simulink model "simulink_computer_auto_highlighted"  (R2022b)
settings: Solver=VariableStepAuto  StartTime=0.0  StopTime=inf  RelTol=1e-3
libraries: simulink_extras x21, dspswit3 x1, simulink x1, hdlsllib x1
(part 2 of 2)

== system simulink_computer_auto_highlighted/Subsystem/Subsystem1/Subsystem3 ==
  In1 : Inport
  In2 : Inport  Port=2
  In3 : Inport  Port=3
  AND : Logic  IconShape=distinctive  AllPortsSameDT=off  OutDataTypeStr=boolean
  AND1 : Logic  IconShape=distinctive  AllPortsSameDT=off  OutDataTypeStr=boolean
  OR : Logic  Operator=OR  IconShape=distinctive  AllPortsSameDT=off  OutDataTypeStr=boolean
  XOR : Logic  Operator=XOR  IconShape=distinctive  AllPortsSameDT=off  OutDataTypeStr=boolean
  XOR1 : Logic  Operator=XOR  IconShape=distinctive  AllPortsSameDT=off  OutDataTypeStr=boolean
  Out1 : Outport
  Out2 : Outport  Port=2
  wires:
  AND1/1 -> OR/1
  AND/1 -> OR/2
  In3/1 -> AND/2, XOR/2
  In2/1 -> AND/1, XOR/1
  In1/1 -> XOR1/2, AND1/2
  XOR/1 -> AND1/1, XOR1/1
  XOR1/1 -> Out1/1
  OR/1 -> Out2/1

== system simulink_computer_auto_highlighted/Subsystem/Subsystem1/Subsystem5 ==
  In1 : Inport
  In2 : Inport  Port=2
  In3 : Inport  Port=3
  AND : Logic  IconShape=distinctive  AllPortsSameDT=off  OutDataTypeStr=boolean
  AND1 : Logic  IconShape=distinctive  AllPortsSameDT=off  OutDataTypeStr=boolean
  OR : Logic  Operator=OR  IconShape=distinctive  AllPortsSameDT=off  OutDataTypeStr=boolean
  XOR : Logic  Operator=XOR  IconShape=distinctive  AllPortsSameDT=off  OutDataTypeStr=boolean
  XOR1 : Logic  Operator=XOR  IconShape=distinctive  AllPortsSameDT=off  OutDataTypeStr=boolean
  Out1 : Outport
  Out2 : Outport  Port=2
  wires:
  AND1/1 -> OR/1
  AND/1 -> OR/2
  In3/1 -> AND/2, XOR/2
  In2/1 -> AND/1, XOR/1
  In1/1 -> XOR1/2, AND1/2
  XOR/1 -> AND1/1, XOR1/1
  XOR1/1 -> Out1/1
  OR/1 -> Out2/1

== matlab function simulink_computer_auto_highlighted/Subsystem1/MATLAB Function ==
  data: b3 input; y output; b2 input; b1 input; b0 input
function y = fcn( b3   , b2   , b1    , b0    )
y =  b3*2^3 + b2*2^2 + b1*2^1 + b0*2^0 ;
end

== matlab function simulink_computer_auto_highlighted/Subsystem8/Subsystem1/MATLAB Function ==
  data: b3 input; y output; b2 input; b1 input; b0 input
function y = fcn( b3   , b2   , b1    , b0    )
y =  b3*2^3 + b2*2^2 + b1*2^1 + b0*2^0 ;
end
